simulink library "DiagM_Lib"  (R2017b)
settings: Solver=VariableStepAuto  StartTime=0.0  StopTime=10.0  RelTol=1e-3
undefined symbols (not defined in the file): StDemErr
libraries: simulink x1
settings Model: Creator=raoy  LastModifiedBy=Raoy

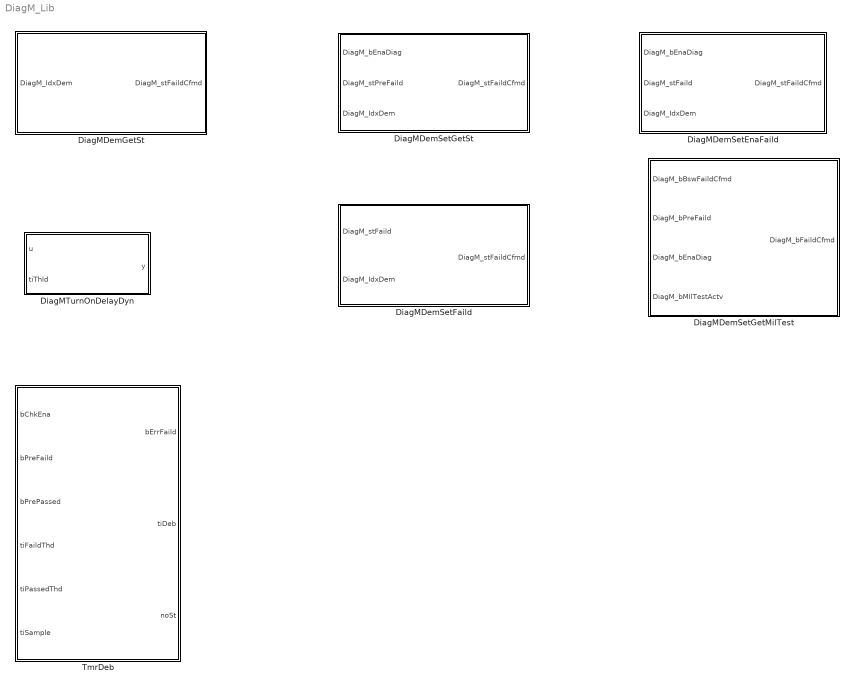
== system DiagM_Lib ==
  DiagMDemGetSt : Subsystem  TreatAsAtomicUnit=on  RTWFcnName=DiagMDemGetSt
      settings: RTWFcnNameOpts=User specified
  DiagMDemSetEnaFaild : Subsystem  TreatAsAtomicUnit=on  RTWFcnName=DiagMDemSetEnaFaild
      settings: RTWFcnNameOpts=User specified
  DiagMDemSetFaild : Subsystem  TreatAsAtomicUnit=on  RTWFcnName=DiagMDemSetFaild
      settings: RTWFcnNameOpts=User specified
  DiagMDemSetGetMilTest : Subsystem  TreatAsAtomicUnit=on  RTWFcnName=DiagMDemSetGetMilTest$C
      settings: RTWFcnNameOpts=User specified
  DiagMDemSetGetSt : Subsystem  TreatAsAtomicUnit=on  RTWFcnName=DiagMDemSetGetSt
      settings: RTWFcnNameOpts=User specified
  DiagMTurnOnDelayDyn : Subsystem  TreatAsAtomicUnit=on  RTWFcnName=DiagMTurnOnDelayDyn
      settings: RTWFcnNameOpts=User specified
  TmrDeb : Stateflow chart  TreatAsAtomicUnit=on

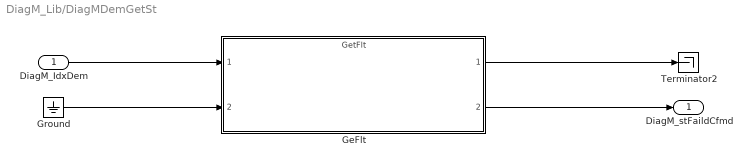
== system DiagM_Lib/DiagMDemGetSt ==
  DiagM_IdxDem : Inport
  GeFlt : ModelReference  ModelNameDialog=GetFlt.slx  SimulationMode=Normal  ModelReferenceVersion=1.3
  Ground : Ground
  Terminator2 : Terminator
  DiagM_stFaildCfmd : Outport  OutDataTypeStr=uint8
  wires:
  Ground/1 -> GeFlt/2
  GeFlt/1 -> Terminator2/1
  DiagM_IdxDem/1 -> GeFlt/1
  GeFlt/2 -> DiagM_stFaildCfmd/1

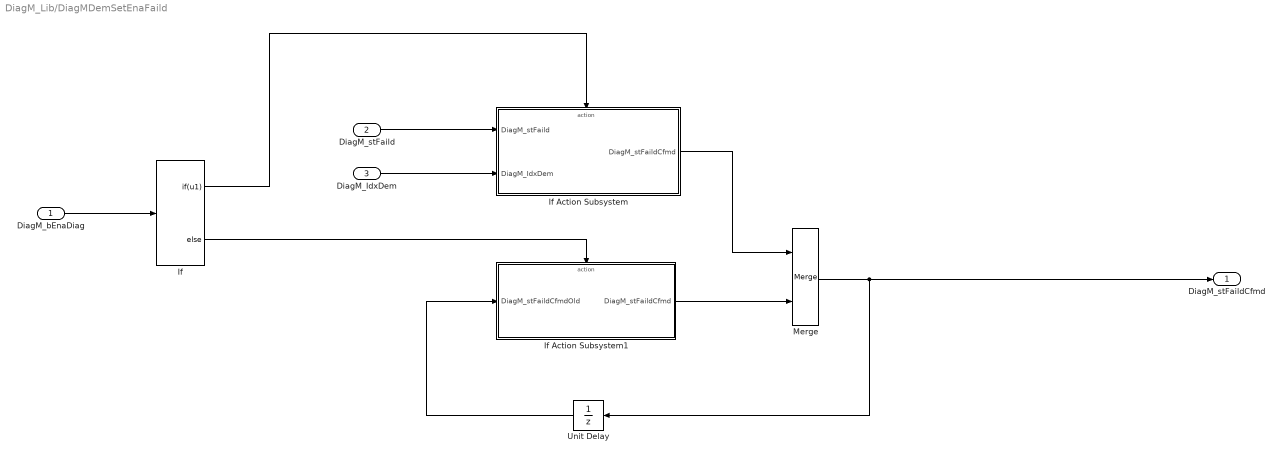
== system DiagM_Lib/DiagMDemSetEnaFaild ==
  DiagM_bEnaDiag : Inport
  DiagM_stFaild : Inport  Port=2
  DiagM_IdxDem : Inport  Port=3
  If : If  IfExpression=u1
  If Action Subsystem : Subsystem  TreatAsAtomicUnit=on
  If Action Subsystem1 : Subsystem  TreatAsAtomicUnit=on
  Merge : Merge
  Unit Delay : UnitDelay  SampleTime=-1
  DiagM_stFaildCfmd : Outport  OutDataTypeStr=uint8
  wires:
  Unit Delay/1 -> If Action Subsystem1/1(DiagM_stFaildCfmdOld)
  Merge/1 -> DiagM_stFaildCfmd/1, Unit Delay/1
  If Action Subsystem1/1(DiagM_stFaildCfmd) -> Merge/2
  If Action Subsystem/1(DiagM_stFaildCfmd) -> Merge/1
  If/2 -> If Action Subsystem1/Action
  DiagM_stFaild/1 -> If Action Subsystem/1(DiagM_stFaild)
  If/1 -> If Action Subsystem/Action
  DiagM_IdxDem/1 -> If Action Subsystem/2(DiagM_IdxDem)
  DiagM_bEnaDiag/1 -> If/1

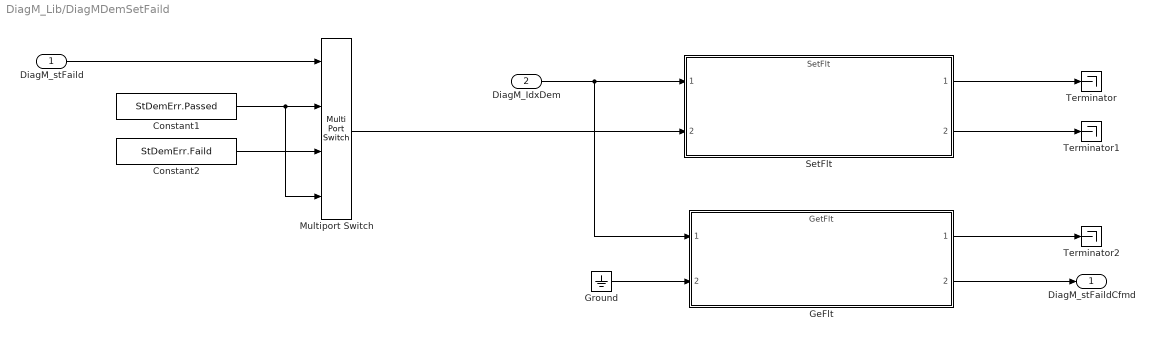
== system DiagM_Lib/DiagMDemSetFaild ==
  DiagM_stFaild : Inport
  DiagM_IdxDem : Inport  Port=2
  Constant1 : Constant  Value=StDemErr.Passed
  Constant2 : Constant  Value=StDemErr.Faild
  GeFlt : ModelReference  ModelNameDialog=GetFlt.slx  SimulationMode=Normal  ModelReferenceVersion=1.3
  Ground : Ground
  Multiport Switch : MultiPortSwitch  DataPortOrder=Zero-based contiguous  Inputs=2  DataPortIndices={0,1}  DataPortForDefault=Additional data port  OutDataTypeStr=Inherit: Inherit via back propagation
  SetFlt : ModelReference  ModelNameDialog=SetFlt.slx  SimulationMode=Normal  ModelReferenceVersion=1.7
  Terminator : Terminator
  Terminator1 : Terminator
  Terminator2 : Terminator
  DiagM_stFaildCfmd : Outport  OutDataTypeStr=uint8
  wires:
  GeFlt/2 -> DiagM_stFaildCfmd/1
  DiagM_IdxDem/1 -> SetFlt/1, GeFlt/1
  SetFlt/2 -> Terminator1/1
  SetFlt/1 -> Terminator/1
  Constant1/1 -> Multiport Switch/4, Multiport Switch/2
  GeFlt/1 -> Terminator2/1
  Ground/1 -> GeFlt/2
  Multiport Switch/1 -> SetFlt/2
  DiagM_stFaild/1 -> Multiport Switch/1
  Constant2/1 -> Multiport Switch/3

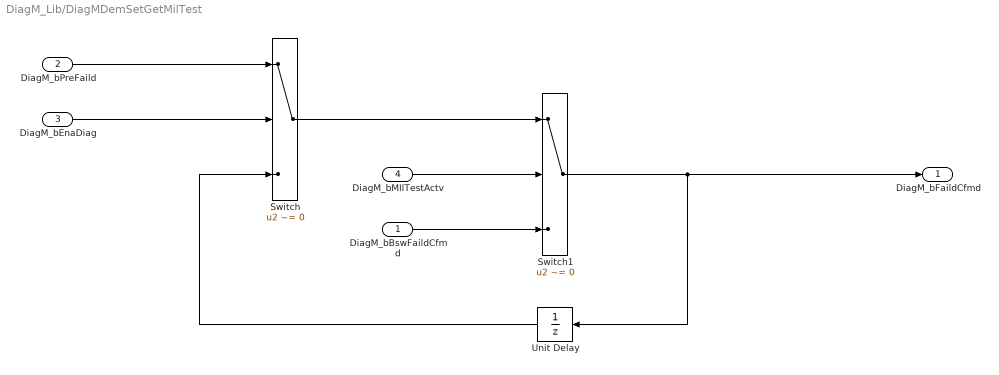
== system DiagM_Lib/DiagMDemSetGetMilTest ==
  DiagM_bBswFaildCfmd : Inport  OutDataTypeStr=boolean
  DiagM_bPreFaild : Inport  Port=2  OutDataTypeStr=boolean
  DiagM_bEnaDiag : Inport  Port=3  OutDataTypeStr=boolean
  DiagM_bMIlTestActv : Inport  Port=4  OutDataTypeStr=boolean
  Switch : Switch  Criteria=u2 ~= 0
  Switch1 : Switch  Criteria=u2 ~= 0
  Unit Delay : UnitDelay  SampleTime=-1
  DiagM_bFaildCfmd : Outport  OutDataTypeStr=boolean
  wires:
  DiagM_bEnaDiag/1 -> Switch/2
  DiagM_bPreFaild/1 -> Switch/1
  DiagM_bMIlTestActv/1 -> Switch1/2
  Switch/1 -> Switch1/1
  Switch1/1 -> Unit Delay/1, DiagM_bFaildCfmd/1
  DiagM_bBswFaildCfmd/1 -> Switch1/3
  Unit Delay/1 -> Switch/3

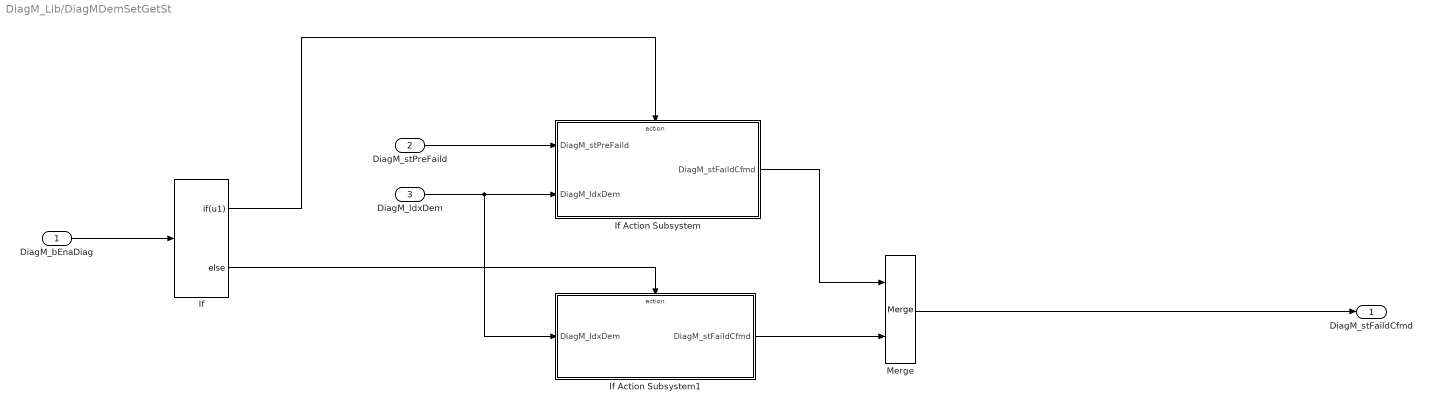
== system DiagM_Lib/DiagMDemSetGetSt ==
  DiagM_bEnaDiag : Inport
  DiagM_stPreFaild : Inport  Port=2
  DiagM_IdxDem : Inport  Port=3
  If : If  IfExpression=u1
  If Action Subsystem : Subsystem  TreatAsAtomicUnit=on
  If Action Subsystem1 : Subsystem  TreatAsAtomicUnit=on
  Merge : Merge
  DiagM_stFaildCfmd : Outport  OutDataTypeStr=uint8
  wires:
  DiagM_bEnaDiag/1 -> If/1
  DiagM_IdxDem/1 -> If Action Subsystem1/1(DiagM_IdxDem), If Action Subsystem/2(DiagM_IdxDem)
  If/1 -> If Action Subsystem/Action
  DiagM_stPreFaild/1 -> If Action Subsystem/1(DiagM_stPreFaild)
  If/2 -> If Action Subsystem1/Action
  If Action Subsystem/1(DiagM_stFaildCfmd) -> Merge/1
  If Action Subsystem1/1(DiagM_stFaildCfmd) -> Merge/2
  Merge/1 -> DiagM_stFaildCfmd/1

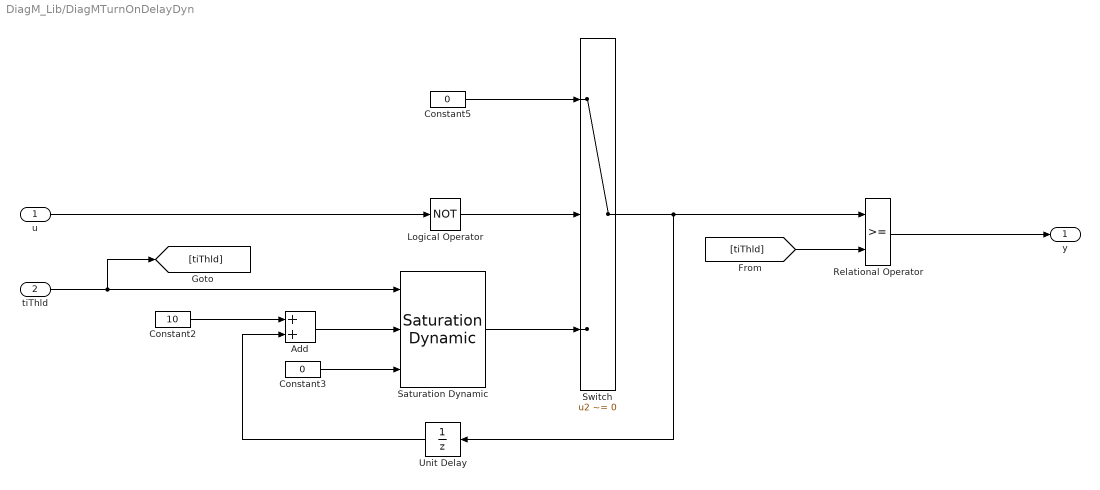
== system DiagM_Lib/DiagMTurnOnDelayDyn ==
  u : Inport  OutDataTypeStr=boolean
  tiThld : Inport  Port=2  OutDataTypeStr=uint16
  Add : Sum
  Constant2 : Constant  Value=10  OutDataTypeStr=uint16
  Constant3 : Constant  Value=0  OutDataTypeStr=uint16
  Constant5 : Constant  Value=0  OutDataTypeStr=uint16
  Logical Operator : Logic  Operator=NOT  AllPortsSameDT=off  OutDataTypeStr=boolean
  Relational Operator : RelationalOperator  OutDataTypeStr=boolean  RndMeth=Simplest
  Saturation Dynamic : simulink/Discontinuities/Saturation Dynamic  OutMin=[]  OutMax=[]  OutDataTypeStr=Inherit: Same as second input  OutDataType=fixdt(1, 16)  OutScaling=2^-10  DoSatur=off
  Switch : Switch  Criteria=u2 ~= 0
  Unit Delay : UnitDelay  SampleTime=-1
  y : Outport
  wires:
  u/1 -> Logical Operator/1
  Switch/1 -> Unit Delay/1, Relational Operator/1
  Unit Delay/1 -> Add/2
  Constant2/1 -> Add/1
  Saturation Dynamic/1 -> Switch/3
  Add/1 -> Saturation Dynamic/2
  Constant3/1 -> Saturation Dynamic/3
  tiThld/1 -> [tiThld], Saturation Dynamic/1
  Relational Operator/1 -> y/1
  Constant5/1 -> Switch/1
  Logical Operator/1 -> Switch/2
  [tiThld] -> Relational Operator/2

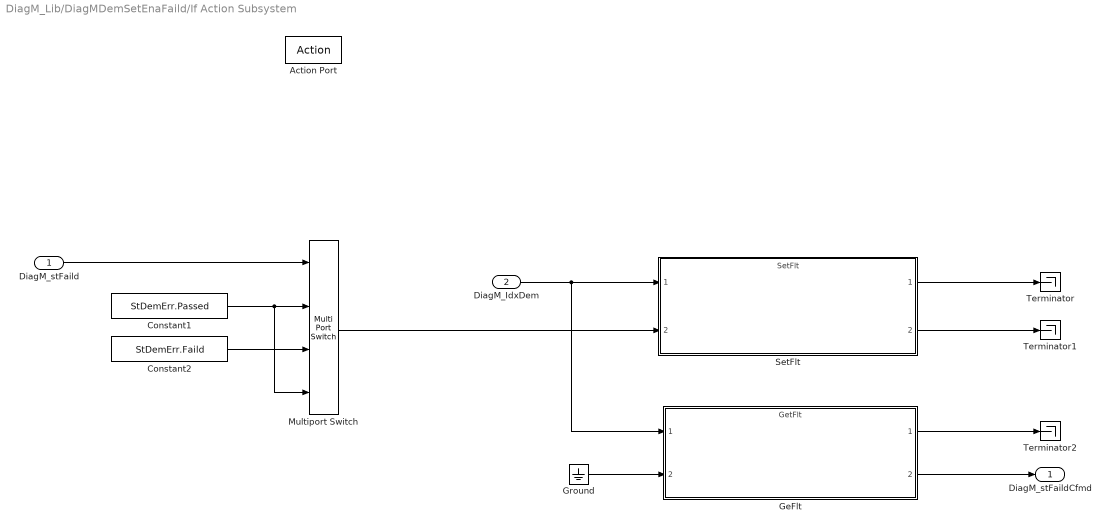
== system DiagM_Lib/DiagMDemSetEnaFaild/If Action Subsystem ==
  DiagM_stFaild : Inport
  DiagM_IdxDem : Inport  Port=2
  Action Port : ActionPort
  Constant1 : Constant  Value=StDemErr.Passed
  Constant2 : Constant  Value=StDemErr.Faild
  GeFlt : ModelReference  ModelNameDialog=GetFlt.slx  SimulationMode=Normal  ModelReferenceVersion=1.3
  Ground : Ground
  Multiport Switch : MultiPortSwitch  DataPortOrder=Zero-based contiguous  Inputs=2  DataPortIndices={0,1}  DataPortForDefault=Additional data port  OutDataTypeStr=Inherit: Inherit via back propagation
  SetFlt : ModelReference  ModelNameDialog=SetFlt.slx  SimulationMode=Normal  ModelReferenceVersion=1.7
  Terminator : Terminator
  Terminator1 : Terminator
  Terminator2 : Terminator
  DiagM_stFaildCfmd : Outport  Description=Parking control status.  OutDataTypeStr=uint8
  wires:
  GeFlt/1 -> Terminator2/1
  Ground/1 -> GeFlt/2
  SetFlt/2 -> Terminator1/1
  SetFlt/1 -> Terminator/1
  DiagM_IdxDem/1 -> GeFlt/1, SetFlt/1
  Multiport Switch/1 -> SetFlt/2
  Constant1/1 -> Multiport Switch/2, Multiport Switch/4
  Constant2/1 -> Multiport Switch/3
  GeFlt/2 -> DiagM_stFaildCfmd/1
  DiagM_stFaild/1 -> Multiport Switch/1

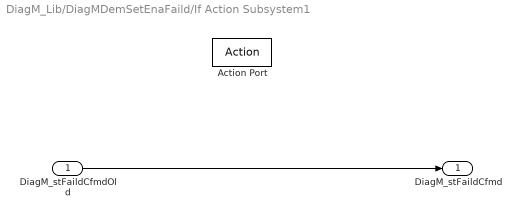
== system DiagM_Lib/DiagMDemSetEnaFaild/If Action Subsystem1 ==
  DiagM_stFaildCfmdOld : Inport
  Action Port : ActionPort
  DiagM_stFaildCfmd : Outport  Description=Parking control status.  OutDataTypeStr=uint8
  wires:
  DiagM_stFaildCfmdOld/1 -> DiagM_stFaildCfmd/1

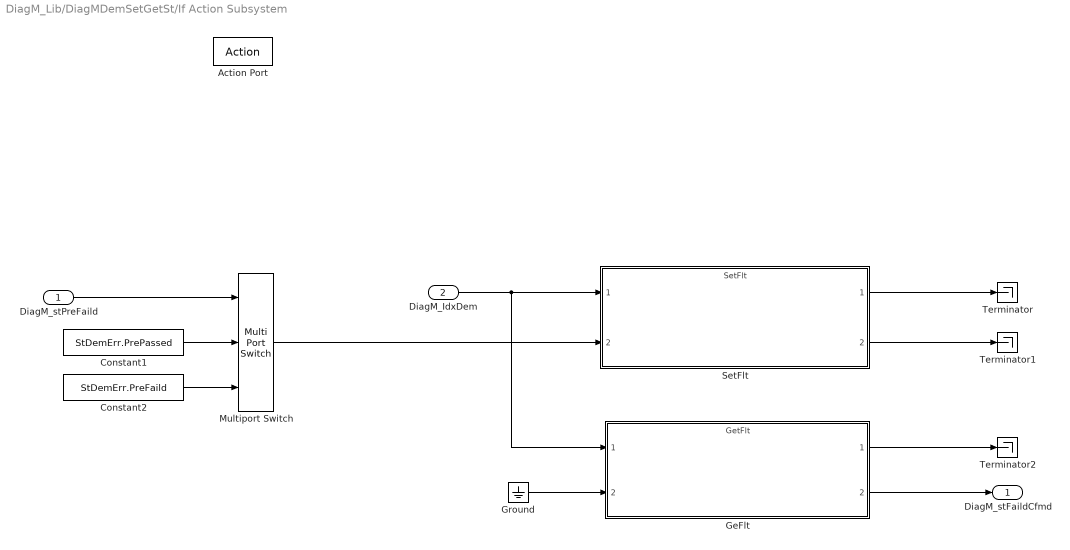
== system DiagM_Lib/DiagMDemSetGetSt/If Action Subsystem ==
  DiagM_stPreFaild : Inport
  DiagM_IdxDem : Inport  Port=2
  Action Port : ActionPort
  Constant1 : Constant  Value=StDemErr.PrePassed
  Constant2 : Constant  Value=StDemErr.PreFaild
  GeFlt : ModelReference  ModelNameDialog=GetFlt.slx  SimulationMode=Normal  ModelReferenceVersion=1.3
  Ground : Ground
  Multiport Switch : MultiPortSwitch  DataPortOrder=Zero-based contiguous  Inputs=2  OutDataTypeStr=Inherit: Inherit via back propagation
  SetFlt : ModelReference  ModelNameDialog=SetFlt.slx  SimulationMode=Normal  ModelReferenceVersion=1.7
  Terminator : Terminator
  Terminator1 : Terminator
  Terminator2 : Terminator
  DiagM_stFaildCfmd : Outport  Description=Parking control status.  OutDataTypeStr=uint8
  wires:
  DiagM_stPreFaild/1 -> Multiport Switch/1
  GeFlt/2 -> DiagM_stFaildCfmd/1
  Constant2/1 -> Multiport Switch/3
  Constant1/1 -> Multiport Switch/2
  Multiport Switch/1 -> SetFlt/2
  DiagM_IdxDem/1 -> SetFlt/1, GeFlt/1
  SetFlt/1 -> Terminator/1
  SetFlt/2 -> Terminator1/1
  Ground/1 -> GeFlt/2
  GeFlt/1 -> Terminator2/1

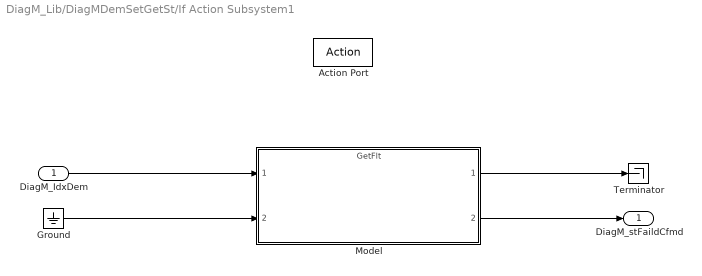
== system DiagM_Lib/DiagMDemSetGetSt/If Action Subsystem1 ==
  DiagM_IdxDem : Inport
  Action Port : ActionPort
  Ground : Ground
  Model : ModelReference  ModelNameDialog=GetFlt.slx  SimulationMode=Normal  ModelReferenceVersion=1.3
  Terminator : Terminator
  DiagM_stFaildCfmd : Outport  Description=Parking control status.  OutDataTypeStr=uint8
  wires:
  Model/2 -> DiagM_stFaildCfmd/1
  Model/1 -> Terminator/1
  Ground/1 -> Model/2
  DiagM_IdxDem/1 -> Model/1

== stateflow chart DiagM_Lib/TmrDeb ==
  state Ini
    en:
    tiDeb=0;
    noSt=1;
    bErrFaild=0;
  state FaildTmr
    en:
    tiDeb=0;
    noSt=2;
    du:
    if (bChkEna&&bPreFaild)
    if (tiDeb>=tiFaildThd)
    bErrFaild=1;
    else
    tiDeb=tiDeb+tiSample;
    end
    else
    tiDeb=0;
    end
  state PassedTmr
    en:
    tiDeb=0;
    noSt=3;
    du:
    if (bChkEna&&bPrePassed)
    if (tiDeb>=tiPassedThd)
    bErrFaild=0;
    else
    tiDeb=tiDeb+tiSample;
    end
    else
    tiDeb=0;
    end
  (default) -> Ini
  Ini -> (junction 8) [order 1] : [bChkEna&&bPreFaild]
  (junction 8) -> FaildTmr
  Ini -> (junction 11) [order 2] : [bChkEna&&bPrePassed]
  (junction 11) -> PassedTmr
  FaildTmr -> PassedTmr : [bChkEna&&bPrePassed]
  PassedTmr -> FaildTmr : [bChkEna&&bPreFaild]
  data: bErrFaild output uint8; bChkEna input; bPreFaild input; bPrePassed input; tiDeb output uint16; tiFaildThd input; tiPassedThd input; tiSample input; noSt output uint8
